simulink model "MotorCC_chopperPWM"  (R2016a)
settings: Solver=ode45  StartTime=0.0  StopTime=0.2  RelTol=1e-3
InitFcn:
  | Tsim = 1;
  | Ra = 0.71218;
  | La = 4.2915e-04;
  | J = 0.00015263;
  | B = 0.00045348;
  | K = 0.072987;
  | TC = 0;
  | Va = 12.4; % Barramento CC %
libraries: powerlib x6, powerlib_meascontrol x2, simulink x1
settings Model: Creator=Lucas Jonys  LastModifiedBy=Lucas Jonys

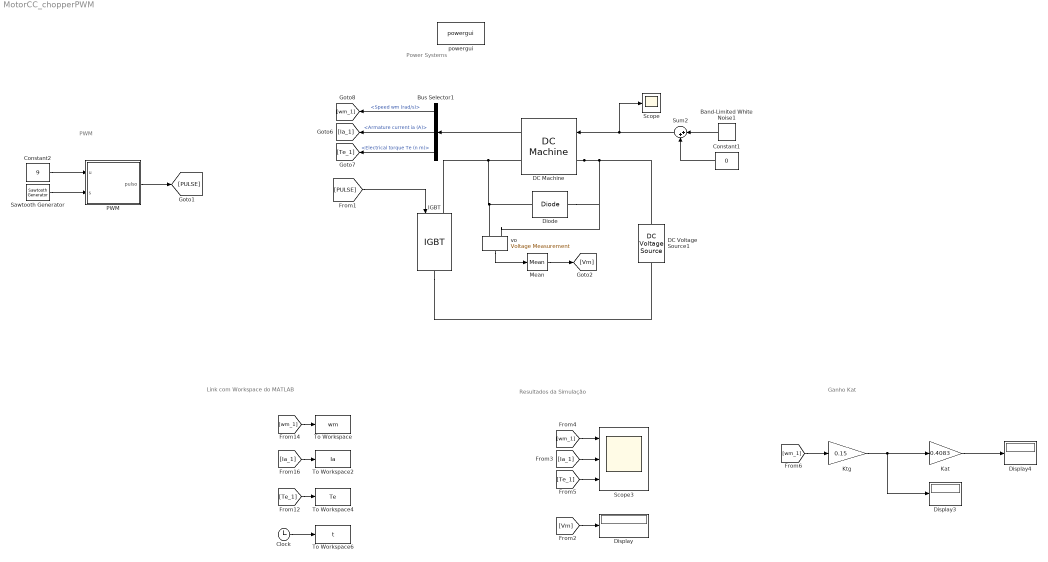
== system MotorCC_chopperPWM ==
  note: Resultados da Simulação
  note: Power Systems
  note: Link com Workspace do MATLAB
  note: PWM
  note: Ganho Kat
  Band-Limited White Noise1 : simulink/Sources/Band-Limited White Noise  Cov=[0.0000001]  Ts=0.0000005  seed=[23341]
  Bus Selector1 : BusSelector  OutputSignals=Speed wm (rad/s),Armature current ia (A),Electrical torque Te (n m)
  Clock : Clock
  Constant1 : Constant  Value=0
  Constant2 : Constant  Value=9
  DC Machine : powerlib/Machines/DC Machine  PresetModel=No  MechanicalLoad=Torque TL  FieldType=Permanent magnet  ShowDetailedParameters=on  MeasurementBus=off  RLa=[Ra La]  RLf="[ 240  120]"  Laf=1.8  MachineConstant=Torque constant (N.m/A)  Ke=1.8  Kt=K  J=J  Bm=B  Tf=TC  w0=0  Ifinit=1  TsPowergui=0  TsBlock=-1
  DC Voltage Source1 : powerlib/Electrical Sources/DC Voltage Source  Amplitude=Va  Measurements=None
  Diode : powerlib/Power Electronics/Diode  Ron=0.15  Lon=0  Vf=0.7  IC=0  UseSnubber=off  Rs=inf  Cs=inf  Measurements=off
  Display : Display
  Display3 : Display
  Display4 : Display
  IGBT : powerlib/Power Electronics/IGBT  Ron=0.01  Lon=0  Vf=0  Tf=1e-6  Tt=2e-6  IC=0  Rs=inf  Cs=inf  Measurements=off
  Kat : Gain  Gain=0.4083
  Ktg : Gain  Gain=0.15
  Mean : powerlib_meascontrol/Measurements/Mean  Freq=4000  Vinit=0  Ts=0
  PWM : Subsystem
  Sawtooth Generator : powerlib_meascontrol/Pulse & Signal Generators/Sawtooth Generator  Freq=4000  Phase=0  Ts=0
  Scope : Scope
  Scope3 : Scope  NumInputPorts=3
  Sum2 : Sum  Inputs=|++
  To Workspace : ToWorkspace  VariableName=wm  SampleTime=-1
  To Workspace2 : ToWorkspace  VariableName=Ia  SampleTime=-1
  To Workspace4 : ToWorkspace  VariableName=Te  SampleTime=-1
  To Workspace6 : ToWorkspace  VariableName=t  SampleTime=-1
  powergui : powerlib/powergui  Priority=1  SimulationMode=Continuous  SolverType=Tustin/Backward Euler (TBE)  SampleTime=50e-6  frequency=60  SPID=on  DisableSnubberDevices=off  DisableRonSwitches=off  DisableVfSwitches=off  SwTol=0  DisplayEquations=off  Interpol=off  ExternalGateDelay=off  methode=off  Ts=100  FunctionMessages=off  echomessages=off  HookPort=off  EnableUseOfTLC=off  x0status=blocks  frequencyindice=0  Pbase=100e6  ErrMax=1e-4  Iterations=50  UnitsV=kV  UnitsW=MW  buscounter=0  RestoreLinks=warning  ResistiveCurrentMeasurement=off  Frange=[0:2:500]  Ylog=off  Xlog=on  ShowGrid=off  save=off  variable=ZData  structure=0  ZoomFFT=off  StartTime=0.0  cycles=1  DisplayStyle=1  fundamental=60  FreqAxis=off  MaxFrequency=1000  frequencyindicesteady=1  RmsSteady=1  display=off
  vo : powerlib/Measurements/Voltage Measurement  PhasorSimulation=off  OutputType=Complex  PSBequivalent=0
  wires:
  [wm_1] -> Scope3/1
  [Te_1] -> Scope3/3
  [Ia_1] -> Scope3/2
  [Te_1] -> To Workspace4/1
  [wm_1] -> To Workspace/1
  [Ia_1] -> To Workspace2/1
  Clock/1 -> To Workspace6/1
  [Vm] -> Display/1
  vo/1 -> Mean/1
  Mean/1 -> [Vm]
  DC Machine/1 -> Bus Selector1/1
  Bus Selector1/1 -> [wm_1]  "<Speed wm (rad/s)>"
  Bus Selector1/2 -> [Ia_1]  "<Armature current ia (A)>"
  Bus Selector1/3 -> [Te_1]  "<Electrical torque Te (n m)>"
  Constant2/1 -> PWM/1(u)
  PWM/1(pulso) -> [PULSE]
  [PULSE] -> IGBT/1
  Sawtooth Generator/1 -> PWM/2(s)
  Constant1/1 -> Sum2/2
  Sum2/1 -> Scope/1, DC Machine/1
  Band-Limited White Noise1/1 -> Sum2/1
  [wm_1] -> Ktg/1
  Ktg/1 -> Kat/1, Display3/1
  Kat/1 -> Display4/1
  connections:
  DC Machine/LConn1 -- Diode/RConn1 -- vo/LConn1 -- DC Voltage Source1/RConn1
  Diode/LConn1 -- vo/LConn2 -- DC Machine/RConn1 -- IGBT/LConn1
  IGBT/RConn1 -- DC Voltage Source1/LConn1

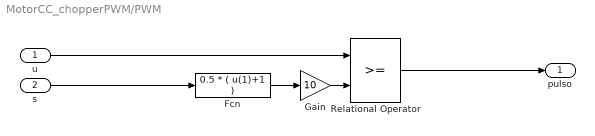
== system MotorCC_chopperPWM/PWM ==
  u : Inport
  s : Inport  Port=2
  Fcn : Fcn  Expr=0.5 * ( u(1)+1 )
  Gain : Gain  Gain=10
  Relational Operator : RelationalOperator  OutDataTypeStr=boolean
  pulso : Outport
  wires:
  Fcn/1 -> Gain/1
  s/1 -> Fcn/1
  Relational Operator/1 -> pulso/1
  u/1 -> Relational Operator/1
  Gain/1 -> Relational Operator/2
